simulink model "LCC_State"  (R2025b)
settings: Solver=FixedStepDiscrete  StartTime=0.0  StopTime=7  FixedStep=.01  RelTol=1e-3
libraries: dspstat3 x1
settings Model: Creator=scb548  LastModifiedBy=scb548
settings OptimizationCC: ZeroExternalMemoryAtStartup=off  ZeroInternalMemoryAtStartup=off
settings RTWCC: SystemTargetFile=rtmaps.tlc  TemplateMakefile=rtmaps_default_tmf  PostCodeGenCommand=rtmaps_post_code_generation(buildInfo)  RetainRTWFile=on  TargetLang=C++  GPUComputeCapability=3.5  Description=Generate an RTMaps component embedding the model
settings STFCustomTargetCC: SystemTargetFile=rtmaps.tlc  TargetLangStandard=C++11 (ISO)  ModelReferenceCompliant=off  CombineOutputUpdateFcns=on  CodeInterfacePackaging=C++ class  SubcomponentCodeInterfacePackaging=C++ class  CPPClassGenCompliant=on  GRTInterface=off  RTMAPS_BOARD=ubuntu2204_x86_64  CustomFileTemplate=rtmaps_file_process.tlc  RTMaps_MultiInstanceCode=1  RTMaps_GRTInterface=0  RTMAPS_ARCH=x86_64  RTMAPS_OS=ubuntu2204  RTMaps_CombineOutputUpdateFcns=1  RTMaps_GenerateAllocFcn=0  DisplayOptimOptions=off  RTMaps_GenerateERTSFunction=0  RTMaps_MatFileLogging=0  RTMaps_IntegerCode=0  RTMAPS_SDKDIR=/opt/rtmaps
settings GRTTargetCC: TargetLangStandard=C++11 (ISO)  ModelReferenceCompliant=off  ParMdlRefBuildCompliant=off  CompOptLevelCompliant=off  MatFileLogging=off  CodeInterfacePackaging=C++ class  SubcomponentCodeInterfacePackaging=C++ class  UseToolchainInfoCompliant=off

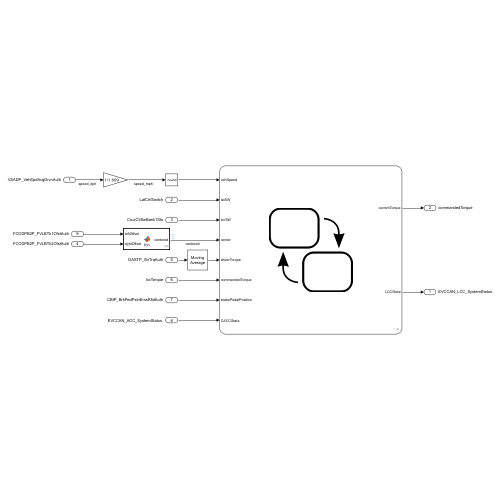
[thumbnail: Simulink's stored preview of the top-level diagram]
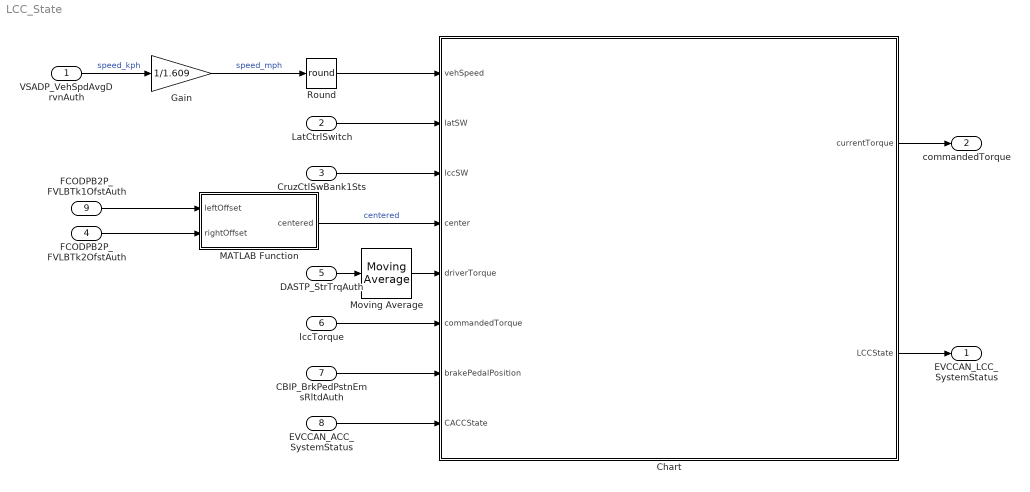
== system LCC_State ==
  VSADP_VehSpdAvgDrvnAuth : Inport  OutDataTypeStr=double
  LatCtrlSwitch : Inport  Port=2  OutDataTypeStr=uint8
  CruzCtlSwBank1Sts : Inport  Port=3  OutDataTypeStr=uint8
  FCODPB2P_FVLBTk2OfstAuth : Inport  Port=4  OutDataTypeStr=double
  DASTP_StrTrqAuth : Inport  Port=5  OutDataTypeStr=double
  lccTorque : Inport  Port=6  OutDataTypeStr=double
  CBIP_BrkPedPstnEmsRltdAuth : Inport  Port=7  OutDataTypeStr=double
  "EVCCAN_ACC_SystemStatus " : Inport  Port=8  OutDataTypeStr=uint8
  FCODPB2P_FVLBTk1OfstAuth : Inport  Port=9  OutDataTypeStr=double
  Chart : Stateflow chart  TreatAsAtomicUnit=on
      settings: PortSchema="{\"entries\":[{\"content\":{\"sides\":[{\"content\":{\"connectorIds\":[\"In1\",\"In7\",\"In8\",\"In4\",\"In6\",\"In5\",\"In3\",\"In2\"]},\"type\":\"ConnectorPlacement.EquallySpacedRectSide\",\"uuid\":\"3024c977-a796-4913-b4ee-7267c2a1ac57\"},{\"content\":{\"connectorIds\":[\"Out1\",\"Out2\"],\"side\":\"RIGHT\"},\"type\":\"ConnectorPlacement.EquallySpacedRectSide\",\"uuid\":\"3a17653d-45a1-48c3-b2d6-ca996b5b4f27\"},{\"content\":{\"side\":\"TOP\"},\"type\":\"ConnectorPlacement.EquallySpacedRectSide\",\"uuid\":\"9e430601-c30b-4fbd-b2ef-51dad258efd7\"}]},\"type\":\"ConnectorPlacement.EquallySpacedConnector\",\"uuid\":\"c142df3b-64bd-48ea-a894-724514be1cd7\"}],\"packageUris\":[\"http://schema.mathworks.com/mf0/Connector/R2020b\"],\"version\":\"1.0\"}"
  Gain : Gain  Gain=1/1.609
  MATLAB Function : MATLAB Function  TreatAsAtomicUnit=on
  Moving Average : dspstat3/Moving Average  Method=Sliding window  ForgettingFactorPort=off  SpecifyWindowLength=on  WindowLength=4  OverlapLength=3  AllowArbitraryInputLength=off  ForgettingFactor=0.9  SimulateUsing=Code generation
  Round : Rounding  Operator=round
  EVCCAN_LCC_SystemStatus : Outport  OutDataTypeStr=uint8  PortDimensions=1
  commandedTorque : Outport  Port=2  OutDataTypeStr=double
  wires:
  VSADP_VehSpdAvgDrvnAuth/1 -> Gain/1  "speed_kph"
  Gain/1 -> Round/1  "speed_mph"
  Round/1 -> Chart/1(vehSpeed)
  Chart/2(LCCState) -> EVCCAN_LCC_SystemStatus/1
  Chart/1(currentTorque) -> commandedTorque/1
  LatCtrlSwitch/1 -> Chart/7(latSW)
  CBIP_BrkPedPstnEmsRltdAuth/1 -> Chart/3(brakePedalPosition)
  lccTorque/1 -> Chart/5(commandedTorque)
  DASTP_StrTrqAuth/1 -> Moving Average/1
  CruzCtlSwBank1Sts/1 -> Chart/8(lccSW)
  FCODPB2P_FVLBTk1OfstAuth/1 -> MATLAB Function/1(leftOffset)
  FCODPB2P_FVLBTk2OfstAuth/1 -> MATLAB Function/2(rightOffset)
  "EVCCAN_ACC_SystemStatus "/1 -> Chart/2(CACCState)
  MATLAB Function/1(centered) -> Chart/4(center)  "centered"
  Moving Average/1 -> Chart/6(driverTorque)

== stateflow chart LCC_State/Chart ==
  state Disabled
    during:
    currentTorque = 0;
    LCCState = 0;
  state ActiveUnpressed
    during:
    currentTorque = commandedTorque;
    LCCState = 2;
  note: CACC State:
      | 0 = Disabled
      | 1 = Standby/Override
      | 2 = Active
      |
      | LCC State:
      | 0 = Disabled (off)
      | 1 = Standby (white)
      | 2 = Active (Green)
      | 3 = Fault (Yellow)
      |
      | CruzCtlSwBank1:
      | 0: No Activation
      | 1: Cancel
      | 2: Cruise on/off
      | 3: Gap
      | 4: LCC Button
      | 5: Lane Departure
      | 6: Short to Ground
      | 7: Short to Power
      | 8: Between Ranges
      | 9: Indeterminate
  state Standby
    during:
    currentTorque = 0;
    LCCState = 1;
  state ActivePressed
    during:
    currentTorque = commandedTorque;
    LCCState = 2;
  (default) -> Disabled
  ActiveUnpressed -> Disabled : [lccSW == 4 || brakePedalPosition>.05 || abs(driverTorque) > abs(commandedTorque) || CACCState ~= 2 || vehSpeed > 35 ]
  Disabled -> Standby : [CACCState==2 && latSW == 1 && center == 1 && vehSpeed <= 35]
  Standby -> Disabled [order 2] : [CACCState ~= 2 || vehSpeed > 35 || brakePedalPosition > .05]
  ActivePressed -> Disabled [order 1] : [brakePedalPosition>.05 || abs(driverTorque) > abs(commandedTorque) || CACCState ~= 2 || vehSpeed > 35 ]
  ActivePressed -> ActiveUnpressed [order 2] : [lccSW == 0]
  Standby -> ActivePressed [order 1] : [lccSW == 4]
  data: currentTorque output double; LCCState output uint8; vehSpeed input double; CACCState input uint8; brakePedalPosition input double; center input double; commandedTorque input double; driverTorque input double; latSW input uint8; lccSW input uint8

== matlab function LCC_State/MATLAB Function ==
  data: leftOffset input; centered output; rightOffset input
function centered = fcn(leftOffset, rightOffset)

    persistent middle
    
    % Avg Left Offset: 1.9m
    % Min Left Offset: -.2m
    % Max Left Offset: 4.7m
    
    if (leftOffset > 2.5 || leftOffset < .5)
        middle = 0;
    
    % Avg Right Offset: -1.8m
    % Min Right Offset: -3.5m
    % Max Right Offset: .2m
    
    elseif (rightOffset < -2.5 || rightOffset > -.5)
        middle = 0;
    
    else
        middle = 1;

    end

    centered = middle;

end
